simulink model "model_gps_unconstr"  (R2019a)
settings: Solver=ode1  StartTime=0.0  StopTime=50  FixedStep=0.01  RelTol=1e-3
libraries: mpclib x1, simulink x1
settings Model: Creator=alexh  LastModifiedBy=alexh
settings DebuggingCC: UnderSpecifiedDimensionMsg=warning

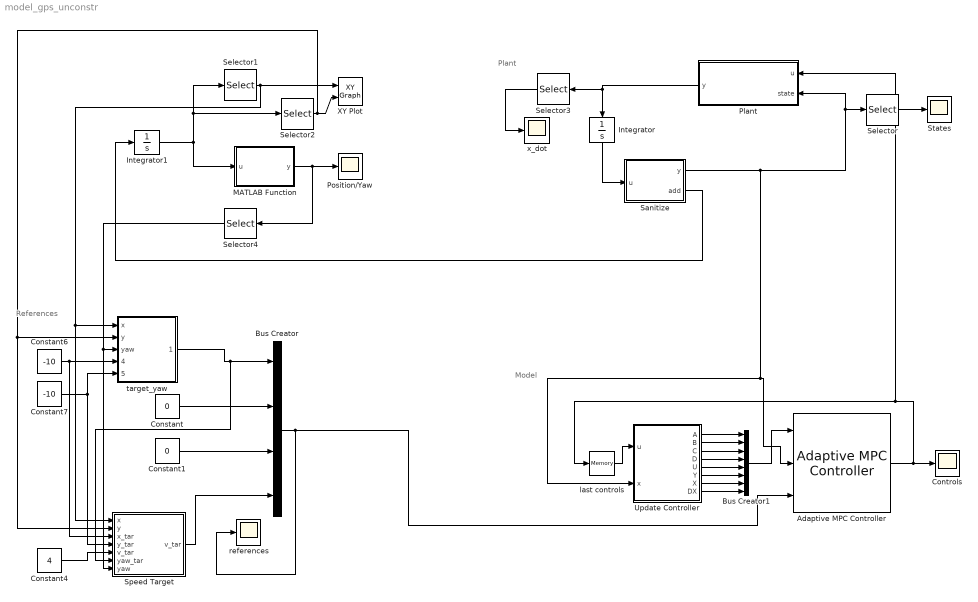
== system model_gps_unconstr ==
  note: Plant
  note: References
  note: Model
  Adaptive MPC Controller : mpclib/Adaptive MPC Controller  SCDEnableBlockLinearizationSpecification=on  mpcobj=mpc_gps_s  enable_value=0  updateMPCinCallerWorkspace=on  md_inport=off  mv_inport=off  uref_inport=off  return_cost=off  return_mvseq=off  return_qpstatus=off  return_xseq=off  return_state=off  return_ovseq=off  state_inport=off  isltv_plant=off  umin_inport=off  umax_inport=off  ymin_inport=off  ymax_inport=off  cc_inport=off  ywt_inport=off  uwt_inport=off  duwt_inport=off  rhoeps_inport=off  pm_inport=off  MaximumP=10  HorizonChoice=FixedHorizon  BlockDataType=double  SampleTimeInherited=off  switch_inport=off
      settings: SourceProductName=MATLAB Runtime - Model Predictive Control Toolbox Addin  SourceProductBaseCode=Missing
  Bus Creator : BusCreator  Inputs=4
  Bus Creator1 : BusCreator  Inputs=8
  Constant : Constant  Value=0
  Constant1 : Constant  Value=0
  Constant4 : Constant  Value=4
  Constant6 : Constant  Value=-10
  Constant7 : Constant  Value=-10
  Controls : Scope
  Integrator : Integrator  InitialCondition=[0;0;0;2]
  Integrator1 : Integrator
  MATLAB Function : MATLAB Function  TreatAsAtomicUnit=on
  Plant : MATLAB Function  TreatAsAtomicUnit=on
  Position/Yaw : Scope
  Sanitize : MATLAB Function  TreatAsAtomicUnit=on
  Selector : Selector  InputPortWidth=4  IndexOptions=Index vector (dialog)  Indices=[1 2 3 4]  OutputSizes=1
  Selector1 : Selector  InputPortWidth=3  IndexOptions=Index vector (dialog)  Indices=[1]  OutputSizes=1
  Selector2 : Selector  InputPortWidth=3  IndexOptions=Index vector (dialog)  Indices=[2]  OutputSizes=1
  Selector3 : Selector  InputPortWidth=4  IndexOptions=Index vector (dialog)  Indices=[1 2 3 4]  OutputSizes=1
  Selector4 : Selector  InputPortWidth=3  IndexOptions=Index vector (dialog)  Indices=[3]  OutputSizes=1
  Speed Target : MATLAB Function  TreatAsAtomicUnit=on
  States : Scope
  Update Controller : MATLAB Function  TreatAsAtomicUnit=on
  XY Plot : simulink/Sinks/XY Graph  xmin=-20  xmax=20  ymin=-20  ymax=20  st=-1
  last controls : Memory  InitialCondition=[0; 0; 0]
  references : Scope
  target_yaw : MATLAB Function  TreatAsAtomicUnit=on
  x_dot : Scope
  wires:
  Constant/1 -> Bus Creator/2
  Constant1/1 -> Bus Creator/3
  Bus Creator/1 -> Adaptive MPC Controller/3, references/1
  Plant/1(y) -> Integrator/1, Selector3/1
  target_yaw/1(yaw_target) -> Speed Target/6(yaw_tar), Bus Creator/1
  Integrator1/1 -> Selector1/1, Selector2/1, MATLAB Function/1(u)
  Selector1/1 -> XY Plot/1, target_yaw/1(x), Speed Target/1(x)
  Selector2/1 -> XY Plot/2, target_yaw/2(y), Speed Target/2(y)
  Sanitize/2(add) -> Integrator1/1
  Constant4/1 -> Speed Target/5("v_tar ")
  Update Controller/1(A) -> Bus Creator1/1
  Update Controller/2(B) -> Bus Creator1/2
  Update Controller/3(C) -> Bus Creator1/3
  Update Controller/4(D) -> Bus Creator1/4
  Update Controller/5(U) -> Bus Creator1/5
  Update Controller/6(Y) -> Bus Creator1/6
  Update Controller/7(X) -> Bus Creator1/7
  Update Controller/8(DX) -> Bus Creator1/8
  Bus Creator1/1 -> Adaptive MPC Controller/1
  last controls/1 -> Update Controller/1(u)
  MATLAB Function/1(y) -> Selector4/1, Position/Yaw/1
  Constant6/1 -> Speed Target/3(x_tar), target_yaw/4(x_target)
  Constant7/1 -> Speed Target/4(y_tar), target_yaw/5(y_target)
  Speed Target/1(v_tar) -> Bus Creator/4
  Adaptive MPC Controller/1 -> Plant/1(u), last controls/1, Controls/1
  Sanitize/1(y) -> Adaptive MPC Controller/2, Update Controller/2(x), Selector/1, Plant/2(state)
  Selector3/1 -> x_dot/1
  Selector/1 -> States/1
  Integrator/1 -> Sanitize/1(u)
  Selector4/1 -> Speed Target/7(yaw), target_yaw/3(yaw)

== matlab function model_gps_unconstr/Sanitize ==
  data: u input; y output; add output
function [y, add]= fcn(u)

y = u;

Vx = u(4);
add = [cos(y(1))*Vx; sin(y(1))*Vx; y(2)];

== matlab function model_gps_unconstr/Plant ==
  data: u input; y output; state input
function y = fcn(u, state)

m = 30;     % Mass
lf = 0.7;   % Distance mass center/front wheel
lr = 0.3;   % Distance mass center/rear wheel
cf = 3000;   % Cornering Stiffness front
cr = 3000;   % Cornering Stiffness rear
iz = 100;   % Yaw Moment of Innertia

Vx = max(2, state(4));

% Continuous-time model
Ac = [0, 1, 0, 0;
       0, -(cr*lr^2+cf*lf^2)/(iz*Vx), -(cr*lr-cf*lf)/iz, 0;
       0, 1-(cr*lr-cf*lf)/(m*Vx^2), -(cf+cr)/(m*Vx), 0;
       0, 0, 0, -1/10];
       
Bc = [0, cf*lf/iz, -cf/(m*Vx), 0;
      0, 0, 0, 1;
      0, 0, 0, -2]';

y = Ac*state + Bc*u;

== matlab function model_gps_unconstr/target_yaw ==
  data: x input; y input; yaw input; yaw_target output; x_target input; y_target input
function yaw_target = fcn(x, y, yaw, x_target, y_target)

% Calculate target yaw
yaw_target = atan2(y_target-y, x_target-x);

% Adjust so we actually take shortest doff
yaw_diff = abs(yaw - yaw_target);

if yaw_diff < pi
    if yaw_target < 0 && yaw > 0
        yaw_target = yaw_target + 2*pi;
    end
    if yaw_target > 0 && yaw < 0
        yaw_target = yaw_target - 2*pi;
    end    
end

== matlab function model_gps_unconstr/Update Controller ==
  data: u input; A output; x input; B output; C output; D output; U output; Y output; X output; DX output
function [A,B,C,D,U,Y,X,DX] = fcn(u,x)

Vx = x(4);

m = 30;     % Mass
lf = 0.7;   % Distance mass center/front wheel
lr = 0.3;   % Distance mass center/rear wheel
cf = 3000;   % Cornering Stiffness front
cr = 3000;   % Cornering Stiffness rear
iz = 100;   % Yaw Moment of Innertia

Ts = 0.01;

if (Vx<2)
       Vx = 2;
end

% Continuous-time model
Ac = [0, 1, 0, 0;
       0, -(cr*lr^2+cf*lf^2)/(iz*Vx), -(cr*lr-cf*lf)/iz, 0;
       0, 1-(cr*lr-cf*lf)/(m*Vx^2), -(cf+cr)/(m*Vx), 0;
       0, 0, 0, -1/10];
       
Bc = [0, cf*lf/iz, -cf/(m*Vx), 0;
      0, 0, 0, 1;
      0, 0, 0, -2]';
 
% Position, Yaw, Speed
Cc = eye(4);
    
Dc = zeros(4, 3);

% Generate discrete-time model
nx = size(Ac,1);
nu = size(Bc,2);
M = expm([[Ac Bc]*Ts; zeros(nu, nx+nu)]);
A = M(1:nx, 1:nx);
A = M(1:nx, 1:nx);
B = M(1:nx, nx+1:nx+nu);
C = Cc;
D = Dc;

X = x';
U = u';
Y = (C*x + D*u)';
DX = (A*x + B*u - x)';

== matlab function model_gps_unconstr/MATLAB Function ==
  data: u input; y output
function y = fcn(u)

yaw_off = u(3)-pi;
u(3) = mod(abs(yaw_off), 2*pi) * sign(yaw_off) + pi;

y = u;

== matlab function model_gps_unconstr/Speed Target ==
  data: x input; y input; v_tar output; x_tar input; y_tar input; v_tar input; yaw_tar input; yaw input
function v_tar = fcn(x, y, x_tar, y_tar, v_tar, yaw_tar, yaw)

% Rearange data
position = [x, y];
position_target = [x_tar, y_tar];

% Calculate delta position
delta_position = position - position_target;
distance_speed = norm(delta_position)/2;
yaw_speed = (v_tar-3*abs(yaw_tar-yaw))+1.5;
current_approp_speed = min(distance_speed, yaw_speed);

v_tar = min(v_tar, current_approp_speed);
